simulink model "pid3"  (R2016a)
settings: Solver=VariableStepAuto  StartTime=0.0  StopTime=10.0  FixedStep=0.01  RelTol=1e-3
libraries: simulink x1
settings Model: Creator=wdj  LastModifiedBy=Mor
settings OptimizationCC: UseFloatMulNetSlope=on
settings DebuggingCC: SFUnexpectedBacktrackingDiag=error  SFNoUnconditionalDefaultTransitionDiag=error
settings GRTTargetCC: TargetLangStandard=C99 (ISO)  GeneratePreprocessorConditionals=Use local settings
settings ConfigComp: CovMetricSettings=dwe  CovHtmlReporting=off  CovSaveCumulativeToWorkspaceVar=off  CovSaveSingleToWorkspaceVar=off  CovExternalEMLEnable=on

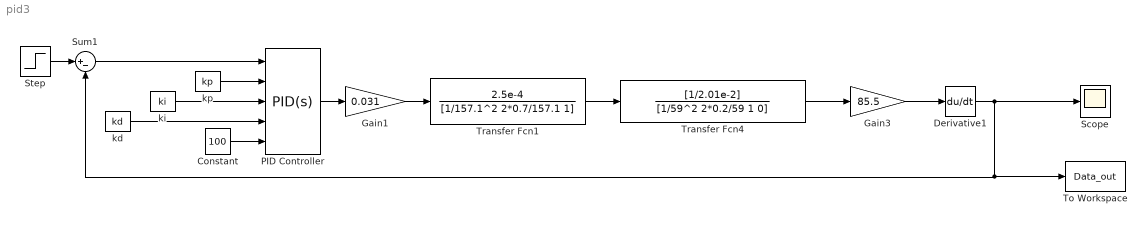
== system pid3 ==
  Constant : Constant  Value=100
  Derivative1 : Derivative
  Gain1 : Gain  Gain=0.031
  Gain3 : Gain  Gain=85.5
  PID Controller : simulink/Continuous/PID Controller  Controller=PID  TimeDomain=Continuous-time  SampleTime=-1  IntegratorMethod=Forward Euler  FilterMethod=Forward Euler  Form=Ideal  UseFilter=on  ControllerParametersSource=external  P=1  I=220  D=0.005  N=100  InitialConditionSource=internal  InitialConditionForIntegrator=0  InitialConditionForFilter=0  ExternalReset=none  LimitOutput=off  UpperSaturationLimit=inf  LowerSaturationLimit=-inf  LinearizeAsGain=on  AntiWindupMode=none  Kb=1  TrackingMode=off  Kt=1  PParamMin=[]  PParamMax=[]  IParamMin=[]  IParamMax=[]  DParamMin=[]  DParamMax=[]  NParamMin=[]  NParamMax=[]  KbParamMin=[]  KbParamMax=[]  KtParamMin=[]  KtParamMax=[]  POutMin=[]  POutMax=[]  IOutMin=[]  IOutMax=[]  DOutMin=[]  DOutMax=[]  NOutMin=[]  NOutMax=[]  KbOutMin=[]  KbOutMax=[]  KtOutMin=[]  KtOutMax=[]  IntegratorOutMin=[]  IntegratorOutMax=[]  FilterOutMin=[]  FilterOutMax=[]  SumOutMin=[]  SumOutMax=[]  SumI1OutMin=[]  SumI1OutMax=[]  SumI2OutMin=[]  SumI2OutMax=[]  SumI3OutMin=[]  SumI3OutMax=[]  SumDOutMin=[]  SumDOutMax=[]  SaturationOutMin=[]  SaturationOutMax=[]  IntegratorContinuousStateAttributes=''  IntegratorStateMustResolveToSignalObject=off  IntegratorRTWStateStorageClass=Auto  FilterContinuousStateAttributes=''  FilterStateMustResolveToSignalObject=off  FilterRTWStateStorageClass=Auto  DifferentiatorICPrevScaledInput=0  DifferentiatorOutMin=[]  DifferentiatorOutMax=[]
  Scope : Scope
  Step : Step  SampleTime=0
  Sum1 : Sum  Inputs=|+-
  To Workspace : ToWorkspace  VariableName=Data_out  SaveFormat=Timeseries  SampleTime=-1
  Transfer Fcn1 : TransferFcn  Numerator=[2.5e-4]  Denominator=[1/157.1^2 2*0.7/157.1 1]
  Transfer Fcn4 : TransferFcn  Numerator=[1/2.01e-2]  Denominator=[1/59^2 2*0.2/59 1 0]
  kd : FromWorkspace  VariableName=kd  SampleTime=0
  ki : FromWorkspace  VariableName=ki  SampleTime=0
  kp : FromWorkspace  VariableName=kp  SampleTime=0
  wires:
  Step/1 -> Sum1/1
  Gain1/1 -> Transfer Fcn1/1
  Transfer Fcn1/1 -> Transfer Fcn4/1
  Transfer Fcn4/1 -> Gain3/1
  Gain3/1 -> Derivative1/1
  Derivative1/1 -> Sum1/2, To Workspace/1, Scope/1
  PID Controller/1 -> Gain1/1
  Sum1/1 -> PID Controller/1
  Constant/1 -> PID Controller/5
  kp/1 -> PID Controller/2
  ki/1 -> PID Controller/3
  kd/1 -> PID Controller/4
